simulink model "Single_quad_Test_paraemeter_010814"  (R2012b)
settings: Solver=ode5  StartTime=0.0  StopTime=inf  FixedStep=sample_time  RelTol=1e-3
InitFcn:
  | sample_time=0.005;%0.004;%0.0025;%0.02;
  | sample_time_Vicon = 0.005;
  | DeltaT = 0.02;
  | g = 9.81;
  | H0 = g%0.3165;
  | Kl = 1;
  | 
  | Q6_mass = 0.8;
  | 
  | Q6_Omega_r = 1.2; %for horizon ref
  | Q6_Zeta_r = 0.707; %for horizon ref
  | Q6_Omega_r_h = 2;%for vertical ref
  | Q6_Zeta_r_h = 0.7; %for vertical ref
  | 
  | 
  | Q6_Omega = 1.5; %for horizon control
  | Q6_Zeta = 0.507; %for horizon control
  | Q6_Omega_h= 2 %for vertical control
  | Q6_Zeta_h = 0.5; %for vertical control
  | 
  | 
  | Q6_acc_max = 5;%horizontal max acc
  | Q6_acc_max_h = 5;%horizontal max acc
  | 
  | omega_h = 0.1;%Ascending speed
  | 
  | MAX_Height = -2;
  | 
  | 
  | % for NN
  | n = 5;
  | r = 3;
  | n2 = 5;
  | NN_ST = 0.02;
  | 
  | GAMA_V = 6;
  | gama_V_e = 0.01;
  | 
  | GAMA_W = GAMA_V;
  | gama_W_e =0.01;
  | 
  | % deadzone
  | NN_Deadzone_Z = 0;
  | 
  | % inputs nomalizaton parameters
  | NN_Z_y_min = -3;
  | NN_Z_y_max = 0.5;
  | 
  | NN_Z_v_max = 8;
  | NN_Z_v_min = -NN_Z_v_max;
  | 
  | % alpha = 0.034;
  | alpha = 1;
  | % c_f = 0.0015;
  | c_f = 0.001;
  | c_y_tilt = 1*0.5;
libraries: X330_Control x5, simulink x2
settings Model: Creator=ttcl3  LastModifiedBy=airshow
settings SolverCC: MaxConsecutiveMinStep=auto
settings DataIOCC: SignalLoggingSaveFormat=ModelDataLogs
settings DebuggingCC: MultiTaskRateTransMsg=warning  FcnCallInpInsideContextMsg=UseLocalSettings
settings SFSimCC: SimParseCustomCode=off
settings GRTTargetCC: CombineOutputUpdateFcns=off  GRTInterface=on

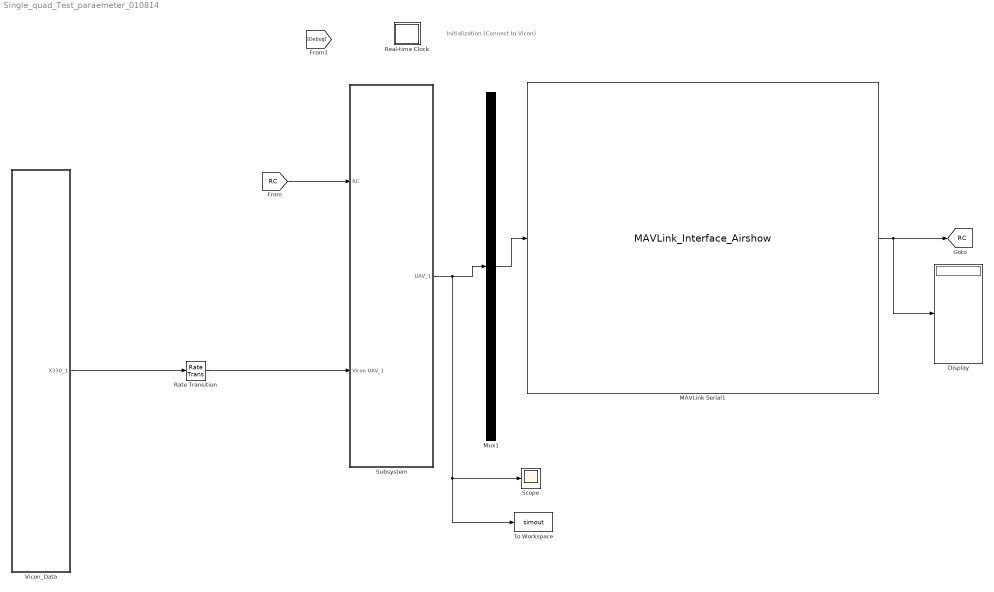
== system Single_quad_Test_paraemeter_010814 ==
  note: Initialization
      | (Connect to Vicon)
  Display : Display
  MAVLink Serial1 : S-Function  FunctionName=MAVLink_Interface_Airshow  Parameters=COM_Port,Baud_Rate,MSG_INPUT,MSG_OUTPUT  EnableBusSupport=off  mask{COM_Port='COM5', Baud_Rate=57600, ATTITUDE_OUT=off, RC_SCALED=on, Quads_1=on, Quads_2=off, Quads_3=off, Quads_4=off, Quads_5=off, Quads_6=off}
      mask prompts: COM_Port "COM Port"; Baud_Rate "Baud Rate"; ATTITUDE_OUT "DEBUG"; RC_SCALED "RC CHANNELS SCALED"; Quads_1 "1 Quad"; Quads_2 "2 Quad"; Quads_3 "3 Quad"; Quads_4 "4 Quad"; Quads_5 "5 Quad"; Quads_6 "6 Quad"
      mask init:
      | MSG_ID_NUM_INPUT = [ uint8(221) uint8(222) uint8(223) uint8(224) uint8(225) uint8(226)];
      | MSG_ID_NAME_INPUT = [Quads_1 Quads_2 Quads_3 Quads_4 Quads_5 Quads_6];
      | 
      | MSG_ID_NUM_OUTPUT = [uint8(34) uint8(30)];
      | MSG_ID_NAME_OUTPUT = [RC_SCALED ATTITUDE_OUT ];
      | 
      | idx_input = find(MSG_ID_NAME_INPUT);
      | MSG_INPUT = MSG_ID_NUM_INPUT(idx_input);
      | 
      | idx_output = find(MSG_ID_NAME_OUTPUT);
      | MSG_OUTPUT = MSG_ID_NUM_OUTPUT(idx_output);
      mask Display:
      | % Block image
      | image(imread('10-inch Quad Heat Map.png'));
      | 
      | %Label block
      | fprintf('MAVLink Serial\n%s\n%dbps', COM_Port,  Baud_Rate)
      | 
      | 
      | %Label input ports
      | 
      | in = 1;
      | if (Quads_1 == 1)
      |     port_label('input', in, 'Quads_1');
      |     in = in + 1;
      | end
      | 
      | if (Quads_2 == 1)
      |     port_label('input', in, 'Quads_2');
      |     in = in + 1;
      | end
      | 
      | if (Quads_3 == 1)
      |     port_label('input', in, 'Quads_3');
      |     in = in + 1;
      | end
      | 
      | if (Quads_4 == 1)
      |     port_label('input', in, 'Quads_4');
      |     in = in + 1;
      | end
      | 
      | if (Quads_5 == 1)
      |     port_label('input', in, 'Quads_5');
      |     in = in + 1;
      | end
      | 
      | 
      | if (Quads_6 == 1)
      |     port_label('input', in, 'Quads_6');
      |     in = in + 1;
      | end
      | %Label output ports
      | 
      | out = 1;
      | if (RC_SCALED == 1)
      |     port_label('output', out, 'RC CMD');
      |     out = out + 1;
      | end
      | 
      | if (ATTITUDE_OUT == 1)
      |     port_label('output', out, 'DEBUG');
      |     out = out + 1;
      | end
  Mux1 : Mux  Inputs=1
  Rate Transition : RateTransition  OutPortSampleTime=0.02
  Real-time Clock : Subsystem  mask(Real-time Clock){sample_time=0.02, tolerance=1}
      mask prompts: sample_time "Synchronize with real-time every n seconds:"; tolerance "Real-time warning tolerance (seconds):"
      mask help: Real-time Synchronization Block
      mask Help: This block synchronizes simulation time with the PC real-time clock or UNIX system clock. The first dialog entry is the period at which the clock is checked to insure real-time synchronization. The second dialog entry is the number of seconds that the simulation time must be within real-time before a warning is printed.
      mask Display: plot(0,0,100,100,[40,60,60,54,54,64,69,76,82,77,81,83,83,81,78,74,70,64,57,49,41,35,32,30,30,31,34,40,47,47,40,40],[90,90,85,85,80,79,76,87,80,70,64,57,49,41,33,28,24,22,21,23,25,31,37,46,56,65,73,78,80,85,85,90],[69,53,53],[64,50,73])
  Scope : Scope
      settings: SaveName=ScopeData2
  Subsystem : Subsystem
  To Workspace : ToWorkspace  VariableName=simout  SampleTime=1  SaveFormat=Structure With Time
  Vicon_Data : Subsystem
  tag scope: RC=global
  wires:
  MAVLink Serial1/1 -> Display/1, [RC]
  Mux1/1 -> MAVLink Serial1/1
  Vicon_Data/1(X330_1) -> Rate Transition/1
  Rate Transition/1 -> Subsystem/2(Vicon UAV_1)
  [RC] -> Subsystem/1(RC)
  Subsystem/1(UAV_1) -> To Workspace/1, Scope/1, Mux1/1

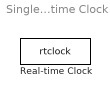
== system Single_quad_Test_paraemeter_010814/Real-time Clock ==
  Real-time Clock : S-Function  FunctionName=rtclock  Parameters=sample_time, tolerance  EnableBusSupport=off

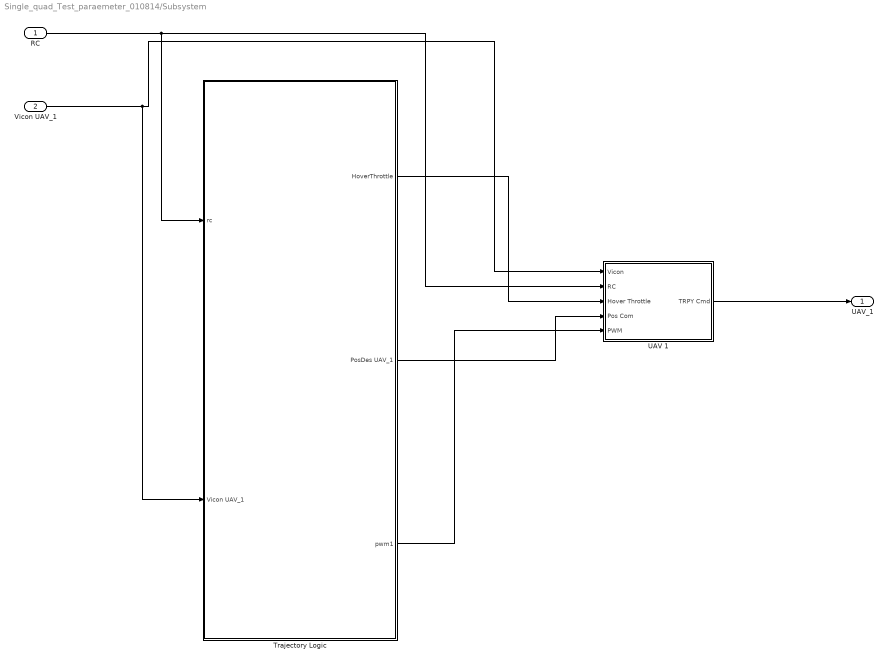
== system Single_quad_Test_paraemeter_010814/Subsystem ==
  RC : Inport
  Vicon UAV_1 : Inport  Port=2
  Trajectory Logic : Subsystem
  UAV 1 : Subsystem
  UAV_1 : Outport
  wires:
  RC/1 -> Trajectory Logic/1(rc), UAV 1/2(RC)
  Vicon UAV_1/1 -> UAV 1/1(Vicon), Trajectory Logic/2(Vicon UAV_1)
  UAV 1/1(TRPY Cmd) -> UAV_1/1
  Trajectory Logic/1(HoverThrottle) -> UAV 1/3(Hover Throttle)
  Trajectory Logic/2(PosDes UAV_1) -> UAV 1/4(Pos Com)
  Trajectory Logic/3(pwm1) -> UAV 1/5(PWM)

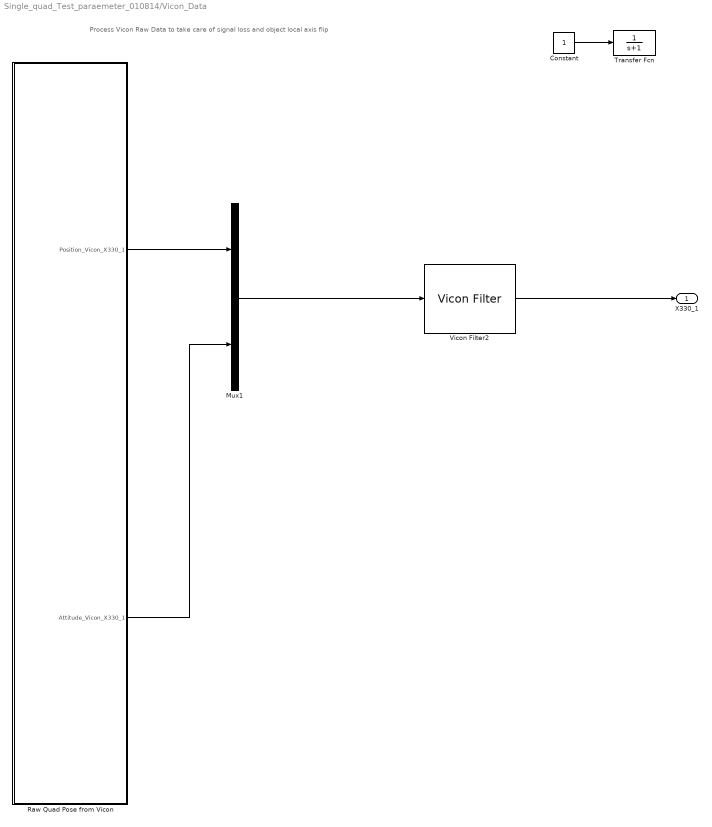
== system Single_quad_Test_paraemeter_010814/Vicon_Data ==
  note: Process Vicon Raw Data to take care of signal loss and object local axis flip
  Constant : Constant  SampleTime=5
  Mux1 : Mux  Inputs=2
  Raw Quad Pose from Vicon : Subsystem
  Transfer Fcn : TransferFcn  Denominator=[1 1]
  Vicon Filter2 : X330_Control/Vicon Filter
  X330_1 : Outport
  wires:
  Vicon Filter2/1 -> X330_1/1
  Constant/1 -> Transfer Fcn/1
  Raw Quad Pose from Vicon/1(Position_Vicon_X330_1) -> Mux1/1
  Raw Quad Pose from Vicon/2(Attitude_Vicon_X330_1) -> Mux1/2
  Mux1/1 -> Vicon Filter2/1

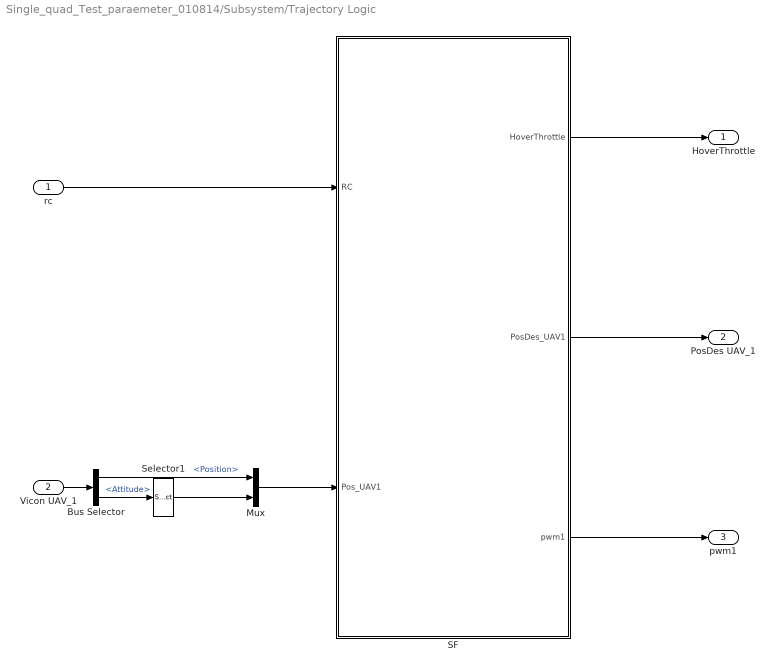
== system Single_quad_Test_paraemeter_010814/Subsystem/Trajectory Logic ==
  rc : Inport
  Vicon UAV_1 : Inport  Port=2
  " SF" : Stateflow chart  TreatAsAtomicUnit=on
  Bus Selector : BusSelector  OutputSignals=Position,Attitude
  Mux : Mux  Inputs=2
  Selector1 : Selector  InputPortWidth=3  IndexOptions=Index vector (dialog)  Indices=[3]  OutputSizes=1
  HoverThrottle : Outport
  PosDes UAV_1 : Outport  Port=2
  pwm1 : Outport  Port=3
  wires:
  Mux/1 -> " SF"/2(Pos_UAV1)
  Selector1/1 -> Mux/2
  Bus Selector/2 -> Selector1/1  "<Attitude>"
  Bus Selector/1 -> Mux/1  "<Position>"
  " SF"/1(HoverThrottle) -> HoverThrottle/1
  rc/1 -> " SF"/1(RC)
  " SF"/2(PosDes_UAV1) -> PosDes UAV_1/1
  Vicon UAV_1/1 -> Bus Selector/1
  " SF"/3(pwm1) -> pwm1/1

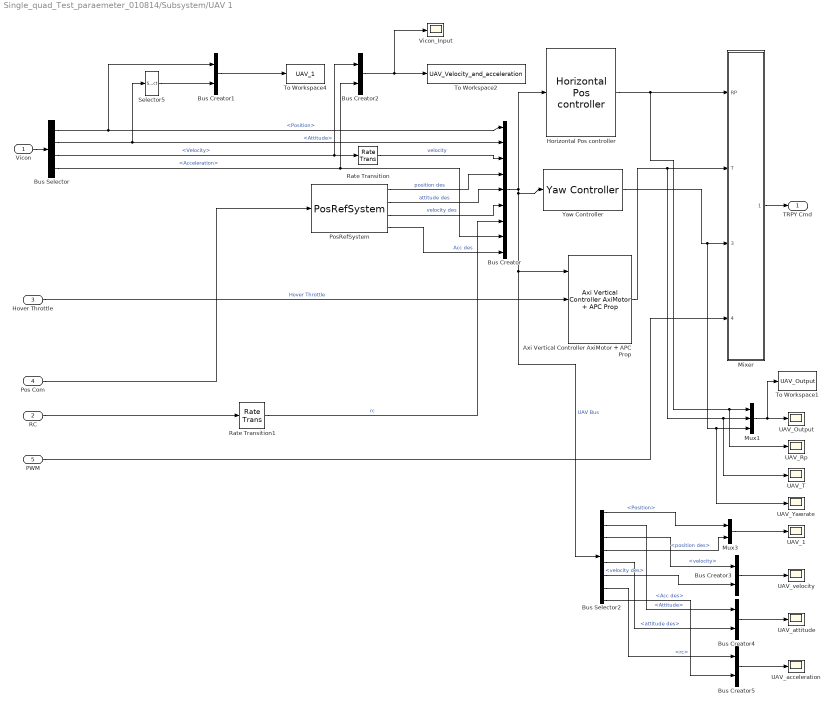
== system Single_quad_Test_paraemeter_010814/Subsystem/UAV 1 ==
  Vicon : Inport
  RC : Inport  Port=2
  Hover Throttle : Inport  Port=3
  Pos Com : Inport  Port=4
  PWM : Inport  Port=5
  Axi Vertical Controller AxiMotor + APC Prop : X330_Control/Axi Vertical Controller AxiMotor + APC Prop  Omega_h=Q6_Omega_h  Zeta_h=Q6_Zeta_h  PID_I_h=1  mass=Q6_mass
  Bus Creator : BusCreator  Inputs=9
  Bus Creator{1..5} (5 alike) : BusCreator  Inputs=2
  Bus Selector : BusSelector  OutputSignals=Position,Attitude,Velocity,Acceleration
  Bus Selector2 : BusSelector  OutputSignals=Position,Attitude,velocity,position des,attitude des,velocity des,rc,Acc des
  Horizontal Pos controller : X330_Control/Horizontal Pos controller  Max_RP=60  Omega=Q6_Omega  PID_i=0.5  Zeta=Q6_Zeta
  Mixer : Subsystem
  Mux1 : Mux  Inputs=3
  Mux3 : Mux  Inputs=2
  PosRefSystem : X330_Control/PosRefSystem  Omega_r=Q6_Omega_r  Zeta_r=Q6_Zeta_r  Acc_Max=Q6_acc_max  Omega_h_r=Q6_Omega_r_h  Zeta_h_r=Q6_Zeta_r_h  Acc_h_Max=Q6_acc_max_h
      link override Saturation: LowerLimit=-3.0
  Rate Transition : RateTransition  OutPortSampleTime=0.02
  Rate Transition1 : RateTransition  OutPortSampleTime=0.02
  Selector5 : Selector  InputPortWidth=3  IndexOptions=Index vector (dialog)  Indices=[3]  OutputSizes=1
  To Workspace1 : ToWorkspace  VariableName=UAV_Output  SampleTime=1  SaveFormat=Structure With Time
  To Workspace2 : ToWorkspace  VariableName=UAV_Velocity_and_acceleration  SampleTime=1  SaveFormat=Structure With Time
  To Workspace4 : ToWorkspace  VariableName=UAV_1  SampleTime=1  SaveFormat=Structure With Time
  UAV_1 : Scope
      settings: TimeRange=10  YMin=-1.75  YMax=0.25
  UAV_Output : Scope
      settings: TimeRange=10  YMin=-1.75  YMax=0.25
  UAV_Rp : Scope
      settings: TimeRange=10  YMin=-1.75  YMax=0.25  SaveName=ScopeData3
  UAV_T : Scope
      settings: TimeRange=10  YMin=-1.75  YMax=0.25  SaveName=ScopeData4
  UAV_Yawrate : Scope
      settings: TimeRange=10  YMin=-1.75  YMax=0.25  SaveName=ScopeData5
  UAV_acceleration : Scope
      settings: ShowLegends=on  TimeRange=10  YMin=-1.75  YMax=0.25  SaveName=ScopeData8
  UAV_attitude : Scope
      settings: TimeRange=10  YMin=-1.75  YMax=0.25  SaveName=ScopeData7
  UAV_velocity : Scope
      settings: TimeRange=10  YMin=-1.75  YMax=0.25  SaveName=ScopeData6
  Vicon_Input : Scope
      settings: TimeRange=10  YMin=-1.75  YMax=0.25  SaveName=ScopeData9
  Yaw Controller : X330_Control/Yaw Controller
  TRPY Cmd : Outport
  wires:
  Mux3/1 -> UAV_1/1
  Bus Selector2/4 -> Mux3/2  "<position des>"
  Bus Selector2/1 -> Mux3/1  "<Position>"
  RC/1 -> Rate Transition1/1
  PosRefSystem/4 -> Bus Creator/9  "Acc des"
  Vicon/1 -> Bus Selector/1
  Bus Selector/3 -> Bus Creator2/1, Rate Transition/1  "<Velocity>"
  Hover Throttle/1 -> Axi Vertical Controller AxiMotor + APC Prop/2  "Hover Throttle"
  PosRefSystem/3 -> Bus Creator/6  "velocity des"
  PosRefSystem/2 -> Bus Creator/5  "attitude des"
  PosRefSystem/1 -> Bus Creator/4  "position des"
  Bus Selector/4 -> Bus Creator2/2, Bus Creator/8  "<Acceleration>"
  Axi Vertical Controller AxiMotor + APC Prop/1 -> UAV_T/1, Mux1/2, Mixer/2(T)
  Yaw Controller/1 -> UAV_Yawrate/1, Mux1/3, Mixer/3(Yaw rate)
  Bus Creator/1 -> Yaw Controller/1, Bus Selector2/1, Axi Vertical Controller AxiMotor + APC Prop/1, Horizontal Pos controller/1  "UAV Bus"
  Rate Transition1/1 -> Bus Creator/7  "rc"
  Rate Transition/1 -> Bus Creator/3  "velocity"
  Horizontal Pos controller/1 -> UAV_Rp/1, Mux1/1, Mixer/1(RP)
  Mixer/1(UAV_1) -> TRPY Cmd/1
  Pos Com/1 -> PosRefSystem/1
  PWM/1 -> Mixer/4(PWM)
  Bus Selector/2 -> Selector5/1, Bus Creator/2  "<Attitude>"
  Bus Selector/1 -> Bus Creator1/1, Bus Creator/1  "<Position>"
  Bus Creator1/1 -> To Workspace4/1
  Selector5/1 -> Bus Creator1/2
  Mux1/1 -> To Workspace1/1, UAV_Output/1
  Bus Creator2/1 -> Vicon_Input/1, To Workspace2/1
  Bus Creator3/1 -> UAV_velocity/1
  Bus Selector2/3 -> Bus Creator3/1  "<velocity>"
  Bus Selector2/6 -> Bus Creator3/2  "<velocity des>"
  Bus Selector2/2 -> Bus Creator4/1  "<Attitude>"
  Bus Selector2/5 -> Bus Creator4/2  "<attitude des>"
  Bus Creator4/1 -> UAV_attitude/1
  Bus Selector2/7 -> Bus Creator5/1  "<rc>"
  Bus Selector2/8 -> Bus Creator5/2  "<Acc des>"
  Bus Creator5/1 -> UAV_acceleration/1

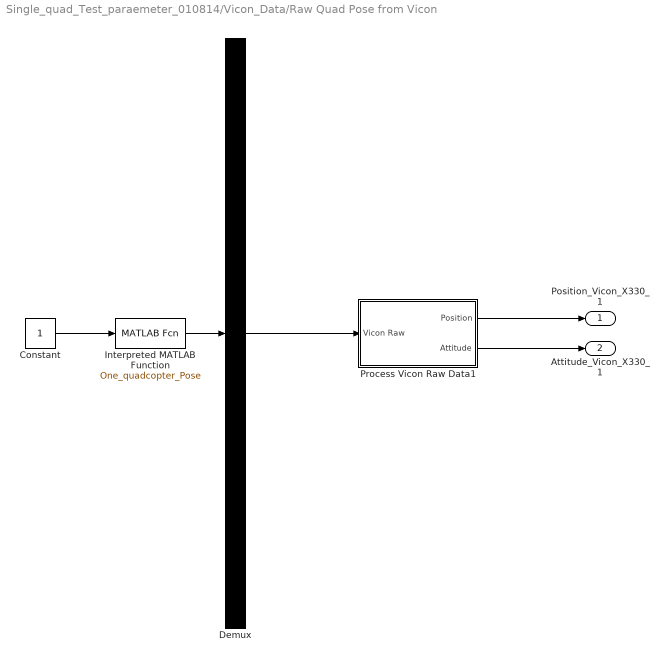
== system Single_quad_Test_paraemeter_010814/Vicon_Data/Raw Quad Pose from Vicon ==
  Constant : Constant  SampleTime=sample_time
  Demux : Demux  Outputs=1
  Interpreted MATLAB Function : MATLABFcn  MATLABFcn=One_quadcopter_Pose
  Process Vicon Raw Data1 : Subsystem
  Position_Vicon_X330_1 : Outport
  Attitude_Vicon_X330_1 : Outport  Port=2
  wires:
  Interpreted MATLAB Function/1 -> Demux/1
  Constant/1 -> Interpreted MATLAB Function/1
  Process Vicon Raw Data1/2(Attitude) -> Attitude_Vicon_X330_1/1
  Process Vicon Raw Data1/1(Position) -> Position_Vicon_X330_1/1
  Demux/1 -> Process Vicon Raw Data1/1(Vicon Raw)

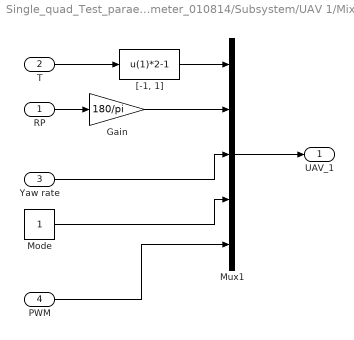
== system Single_quad_Test_paraemeter_010814/Subsystem/UAV 1/Mixer ==
  RP : Inport
  T : Inport  Port=2
  Yaw rate : Inport  Port=3
  PWM : Inport  Port=4
  Gain : Gain  Gain=180/pi
  Mode : Constant  SampleTime=0.02
  Mux1 : Mux  Inputs=5
  "[-1, 1]" : Fcn  Expr=u(1)*2-1
  UAV_1 : Outport
  wires:
  "[-1, 1]"/1 -> Mux1/1
  Gain/1 -> Mux1/2
  Mode/1 -> Mux1/4
  Yaw rate/1 -> Mux1/3
  RP/1 -> Gain/1
  T/1 -> "[-1, 1]"/1
  Mux1/1 -> UAV_1/1
  PWM/1 -> Mux1/5

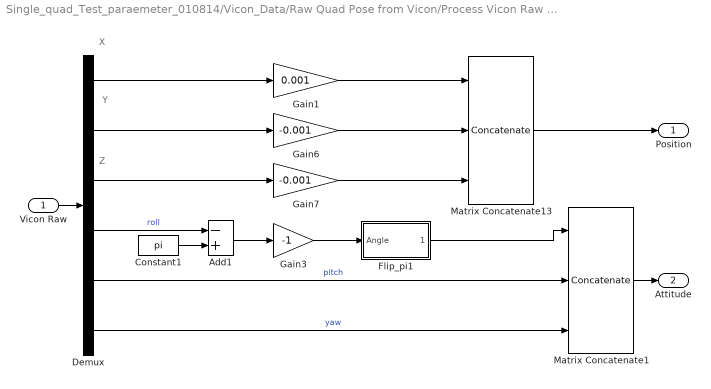
== system Single_quad_Test_paraemeter_010814/Vicon_Data/Raw Quad Pose from Vicon/Process Vicon Raw Data1 ==
  note: X
  note: Y
  note: Z
  Vicon Raw : Inport
  Add1 : Sum  Inputs=-+
  Constant1 : Constant  Value=pi  OutDataTypeStr=double
  Demux : Demux  Outputs=6
  Flip_pi1 : Subsystem  mask(Flip -pi to pi){}
      mask help: Flips the inputs into the range -pi to pi
      mask Help: Flips the inputs into the range -pi to pi
      mask Display: disp('Flip_pi')
  Gain1 : Gain  Gain=0.001
  Gain3 : Gain  Gain=-1
  Gain6 : Gain  Gain=-0.001
  Gain7 : Gain  Gain=-0.001
  Matrix Concatenate1 : Concatenate  NumInputs=3  Mode=Multidimensional array
  Matrix Concatenate13 : Concatenate  NumInputs=3  Mode=Multidimensional array
  Position : Outport
  Attitude : Outport  Port=2
  wires:
  Constant1/1 -> Add1/2
  Demux/6 -> Matrix Concatenate1/3  "yaw"
  Gain1/1 -> Matrix Concatenate13/1
  Demux/1 -> Gain1/1
  Demux/2 -> Gain6/1
  Demux/3 -> Gain7/1
  Demux/4 -> Add1/1  "roll"
  Gain6/1 -> Matrix Concatenate13/2
  Gain7/1 -> Matrix Concatenate13/3
  Add1/1 -> Gain3/1
  Gain3/1 -> Flip_pi1/1(Angle)
  Demux/5 -> Matrix Concatenate1/2  "pitch"
  Flip_pi1/1(Angle_Flip) -> Matrix Concatenate1/1
  Matrix Concatenate13/1 -> Position/1
  Vicon Raw/1 -> Demux/1
  Matrix Concatenate1/1 -> Attitude/1

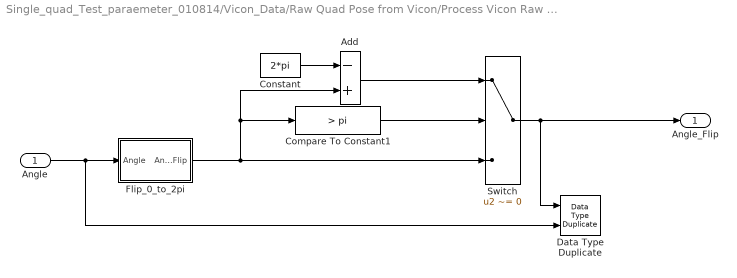
== system Single_quad_Test_paraemeter_010814/Vicon_Data/Raw Quad Pose from Vicon/Process Vicon Raw Data1/Flip_pi1 ==
  Angle : Inport
  Add : Sum  Inputs=-+
  Compare To Constant1 : simulink/Logic and Bit Operations/Compare To Constant  relop=>  const=pi  OutDataTypeStr=uint8  ZeroCross=off
  Constant : Constant  Value=2*pi
  Data Type Duplicate : DataTypeDuplicate
  Flip_0_to_2pi : Subsystem  mask(Flip zero to 2pi){}
      mask help: Flips the inputs into the range zero to +2pi
      mask Help: Flips the inputs into the range zero to +2pi
      mask Display: disp('Flip_0_2pi')
  Switch : Switch  Criteria=u2 ~= 0
  Angle_Flip : Outport
  wires:
  Switch/1 -> Data Type Duplicate/1, Angle_Flip/1
  Add/1 -> Switch/1
  Constant/1 -> Add/1
  Compare To Constant1/1 -> Switch/2
  Flip_0_to_2pi/1(Angle_Flip) -> Add/2, Compare To Constant1/1, Switch/3
  Angle/1 -> Data Type Duplicate/2, Flip_0_to_2pi/1(Angle)

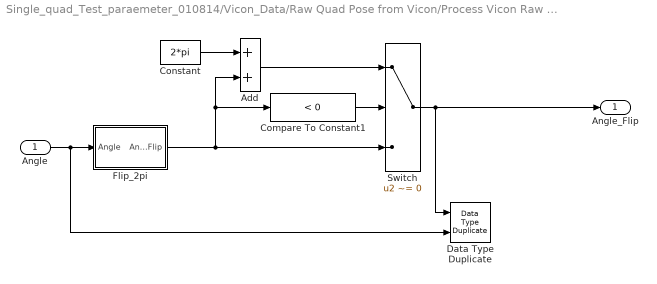
== system Single_quad_Test_paraemeter_010814/Vicon_Data/Raw Quad Pose from Vicon/Process Vicon Raw Data1/Flip_pi1/Flip_0_to_2pi ==
  Angle : Inport
  Add : Sum
  Compare To Constant1 : simulink/Logic and Bit Operations/Compare To Constant  relop=<  const=0  OutDataTypeStr=uint8  ZeroCross=off
  Constant : Constant  Value=2*pi
  Data Type Duplicate : DataTypeDuplicate
  Flip_2pi : Subsystem  mask(Flip -2pi to 2pi){}
      mask help: Flips the inputs into the range -2pi to +2pi
      mask Help: Flips the inputs into the range -2pi to +2pi
      mask Display: disp('Flip_2pi')
  Switch : Switch  Criteria=u2 ~= 0
  Angle_Flip : Outport
  wires:
  Switch/1 -> Data Type Duplicate/1, Angle_Flip/1
  Angle/1 -> Data Type Duplicate/2, Flip_2pi/1(Angle)
  Add/1 -> Switch/1
  Constant/1 -> Add/1
  Compare To Constant1/1 -> Switch/2
  Flip_2pi/1(Angle_Flip) -> Switch/3, Add/2, Compare To Constant1/1

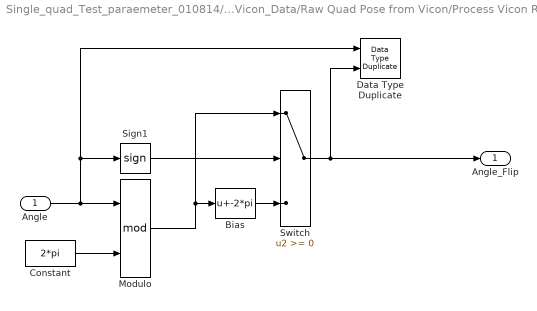
== system Single_quad_Test_paraemeter_010814/Vicon_Data/Raw Quad Pose from Vicon/Process Vicon Raw Data1/Flip_pi1/Flip_0_to_2pi/Flip_2pi ==
  Angle : Inport
  Bias : Bias  Bias=-2*pi
  Constant : Constant  Value=2*pi
  Data Type Duplicate : DataTypeDuplicate
  Modulo : Math  Operator=mod  SaturateOnIntegerOverflow=on
  Sign1 : Signum
  Switch : Switch
  Angle_Flip : Outport
  wires:
  Switch/1 -> Data Type Duplicate/2, Angle_Flip/1
  Bias/1 -> Switch/3
  Sign1/1 -> Switch/2
  Modulo/1 -> Switch/1, Bias/1
  Constant/1 -> Modulo/2
  Angle/1 -> Data Type Duplicate/1, Sign1/1, Modulo/1

== stateflow chart Single_quad_Test_paraemeter_010814/Subsystem/Trajectory Logic/ SF ==
  state Airborne
    state TakeOff
      du:		HoverThrottle = (H0 - HoverThrottle)*2*DeltaT + HoverThrottle ;
      PosDes_UAV1[2] = (-1.2 - PosDes_UAV1[2])*1*DeltaT + PosDes_UAV1[2] ;
      PosDes_UAV1[3] = 0 ;
    state Red_UAV1
      du:PosDes_UAV1[0] = (0- PosDes_UAV1[0])*0.75*DeltaT + PosDes_UAV1[0] ;
      PosDes_UAV1[1] = (0- PosDes_UAV1[1])*0.75*DeltaT + PosDes_UAV1[1] ;
      PosDes_UAV1[2] = (-1.5- PosDes_UAV1[2])*0.75*DeltaT + PosDes_UAV1[2] ;
      PosDes_UAV1[3] = 0 ;
    (default) -> TakeOff : {	PosDes_UAV1 = Pos_UAV1;
        |
        | 	 }
    TakeOff -> Red_UAV1 : after (3, sec)
  state Landing
    state Decsending
      en:		PosDes_UAV1 = Pos_UAV1;
      du:		PosDes_UAV1[2] = (0 - PosDes_UAV1[2])*0.2*DeltaT + PosDes_UAV1[2] ;
    state CutThrottle
      du:		HoverThrottle = (0.0 - HoverThrottle)*3*DeltaT + HoverThrottle ;
    (default) -> Decsending
    Decsending -> (junction 288) : after(2,sec)
    (junction 288) -> CutThrottle : [Pos_UAV1[2] > -0.2]
  Landing -> Airborne : [RC[6] > 0.5]
  Airborne -> Landing : [RC[6] < -0.5]
  (default) -> Landing : {HoverThrottle=0.0}
  data: HoverThrottle output double size=1; PosDes_UAV1 output double size=4; RC input size=8; Pos_UAV1 input size=4; DeltaT parameter size=1; H0 parameter size=1; Kl parameter size=1; omega_h parameter; MAX_Height parameter size=1; pwm1 output double
